simulink model "hw1simq3"  (R2024b)
settings: Solver=ode1  StartTime=0.0  StopTime=20  FixedStep=1/24  RelTol=1e-3
settings Model: Creator=yugpn  LastModifiedBy=JTerr

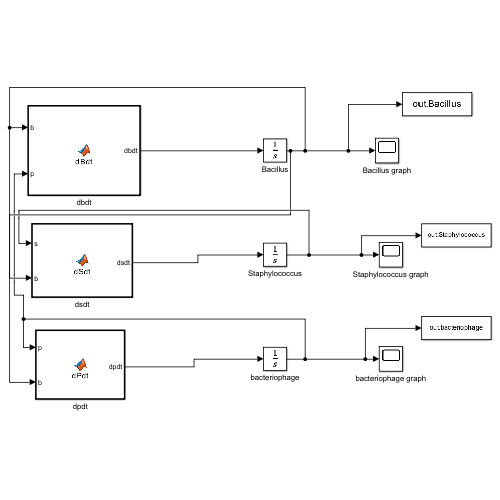
[thumbnail: Simulink's stored preview of the top-level diagram]
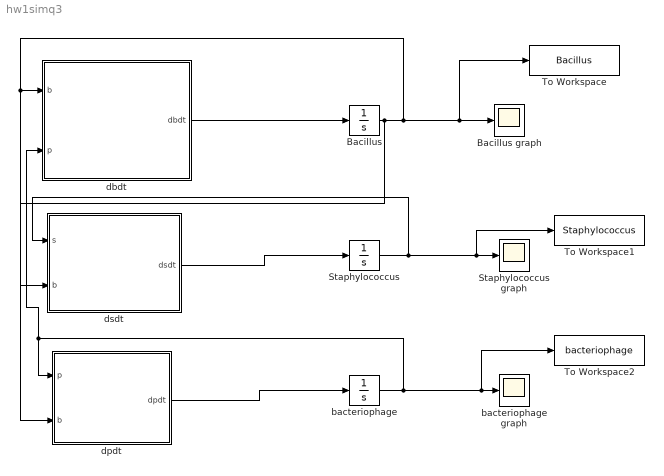
== system hw1simq3 ==
  Bacillus : Integrator  InitialCondition=1e4
  Bacillus graph : Scope
  Staphylococcus : Integrator  InitialCondition=1e4
  Staphylococcus graph : Scope
  To Workspace : ToWorkspace  VariableName=Bacillus  SampleTime=-1
      settings: Save2DSignal=2-D array (concatenate along first dimension)
  To Workspace1 : ToWorkspace  VariableName=Staphylococcus  SampleTime=-1
      settings: Save2DSignal=2-D array (concatenate along first dimension)
  To Workspace2 : ToWorkspace  VariableName=bacteriophage  SampleTime=-1
      settings: Save2DSignal=2-D array (concatenate along first dimension)
  bacteriophage : Integrator  InitialCondition=1e2
  bacteriophage graph : Scope
  dbdt : MATLAB Function  TreatAsAtomicUnit=on
  dpdt : MATLAB Function  TreatAsAtomicUnit=on
  dsdt : MATLAB Function  TreatAsAtomicUnit=on
  wires:
  dbdt/1(dbdt) -> Bacillus/1
  dsdt/1(dsdt) -> Staphylococcus/1
  dpdt/1(dpdt) -> bacteriophage/1
  Bacillus/1 -> dsdt/2(b), dpdt/2(b), dbdt/1(b), To Workspace/1, Bacillus graph/1
  bacteriophage/1 -> dpdt/1(p), dbdt/2(p), To Workspace2/1, bacteriophage graph/1
  Staphylococcus/1 -> dsdt/1(s), To Workspace1/1, Staphylococcus graph/1

== matlab function hw1simq3/dpdt ==
  data: p input; dpdt output; b input
function dpdt = dPdt(p, b)
    % Parameters
    x = 1e-6;
    n = 0.9;
    
    % Differential equation for p
    dpdt = -n * p + x * b * p;
end

== matlab function hw1simq3/dbdt ==
  data: b input; dbdt output; p input
function dbdt = dBdt(b, p)
    % Parameters
    k1 = 1.25;
    CC1 = 1e10;
    x = 1e-6;
    
    % Differential equation for b
    dbdt = k1 * b * (1 - b / CC1) - x * p * b;
end

== matlab function hw1simq3/dsdt ==
  data: s input; dsdt output; b input
function dsdt = dSdt(s, b)
    % Parameters
    k2 = 2.0;
    CC2 = 1e10;
    m = 1.7e4;
    
    % Differential equation for s
    dsdt = k2 * s * (1 - s / CC2) - (m * b / CC2);
end
